simulink model "model"  (R2025b)
settings: Solver=VariableStepAuto  StartTime=0.0  StopTime=50  RelTol=1e-3
values from neighbouring files (symbols this model uses):
  a = 0.1165    [model_init.m]
  b = -3.915    [model_init.m]
  c = -0.008    [model_init.m]
  d = 0.00229    [model_init.m]
  K = lqr(A, B, Q, R)    [model_init.m]
  Km = 484.73    [model_init.m]
  SP = [pi, 0, 0]    [model_init.m]
  x0 = [pi+0.3 ; 0; 0]    [model_init.m]
settings Model: Creator=kamil  LastModifiedBy=kamil

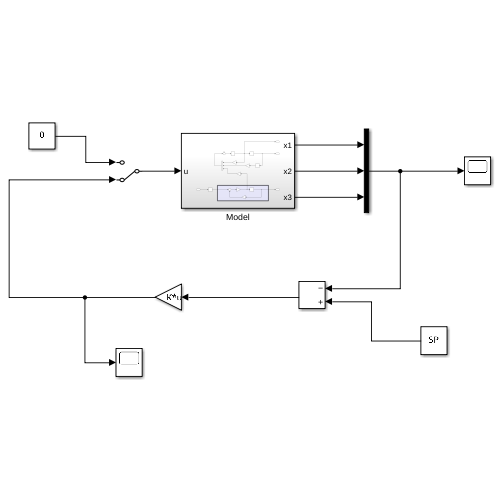
[thumbnail: Simulink's stored preview of the top-level diagram]
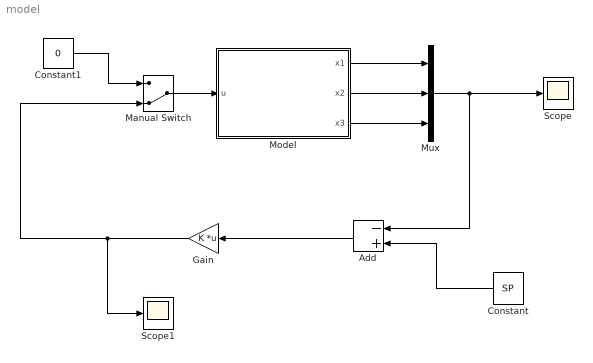
== system model ==
  Add : Sum  Inputs=-+
  Constant : Constant  Value=SP
  Constant1 : Constant  Value=0
  Gain : Gain  Gain=K  Multiplication=Matrix(K*u)
  Manual Switch : ManualSwitch  CurrentSetting=0
  Model : Subsystem
  Mux : Mux  Inputs=3
  Scope : Scope
      settings: ActiveDisplayYMinimum=-5.8513416349939282  ActiveDisplayYMaximum=9.75484977597095
  Scope1 : Scope
      settings: ActiveDisplayYMinimum=-0.14715208233080201  ActiveDisplayYMaximum=3.6607519510349813
  wires:
  Model/1(x1) -> Mux/1
  Model/2(x2) -> Mux/2
  Model/3(x3) -> Mux/3
  Mux/1 -> Scope/1, Add/1
  Constant/1 -> Add/2
  Add/1 -> Gain/1
  Gain/1 -> Manual Switch/2, Scope1/1
  Manual Switch/1 -> Model/1(u)
  Constant1/1 -> Manual Switch/1

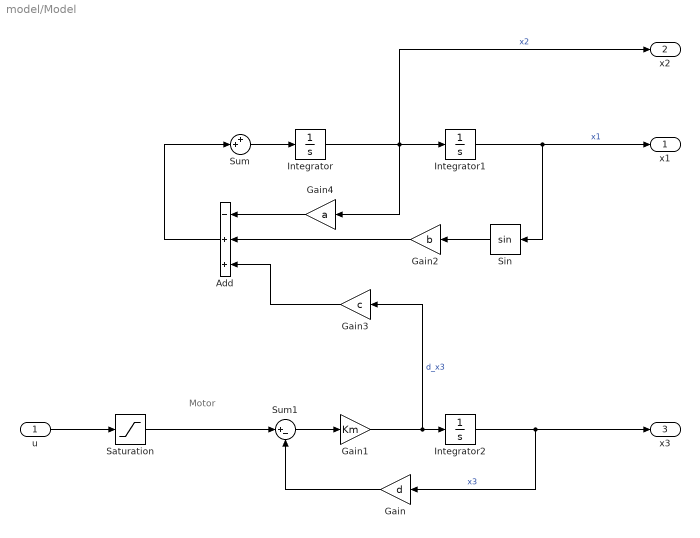
== system model/Model ==
  note: Motor
  u : Inport
  Add : Sum  Inputs=-++
  Gain : Gain  Gain=d
  Gain1 : Gain  Gain=Km
  Gain2 : Gain  Gain=b
  Gain3 : Gain  Gain=c
  Gain4 : Gain  Gain=a
  Integrator : Integrator  InitialCondition=x0(2)
  Integrator1 : Integrator  InitialCondition=x0(1)
  Integrator2 : Integrator  InitialCondition=x0(3)
  Saturation : Saturate  UpperLimit=1  LowerLimit=-1
  Sin : Trigonometry
  Sum : Sum  Inputs=++|
  Sum1 : Sum  Inputs=|+-
  x1 : Outport
  x2 : Outport  Port=2
  x3 : Outport  Port=3
  wires:
  Sin/1 -> Gain2/1
  Gain3/1 -> Add/3
  Sum1/1 -> Gain1/1
  Integrator1/1 -> x1/1, Sin/1  "x1"
  Gain4/1 -> Add/1
  Add/1 -> Sum/2
  Gain2/1 -> Add/2
  Integrator/1 -> x2/1, Integrator1/1, Gain4/1  "x2"
  Gain1/1 -> Gain3/1, Integrator2/1  "d_x3"
  Gain/1 -> Sum1/2
  Integrator2/1 -> x3/1, Gain/1  "x3"
  u/1 -> Saturation/1
  Saturation/1 -> Sum1/1
  Sum/1 -> Integrator/1
